simulink model "inverters_action_ETR07"  (R2017b)
settings: Solver=FixedStepAuto  StartTime=0.0  StopTime=10.0  RelTol=1e-3
libraries: simulink x8
settings Model: Creator=cspt  LastModifiedBy=cspt
settings RTWCC: SystemTargetFile=irt.tlc  TemplateMakefile=irt_default_tmf  Description=INTECRIO Real-Time Target
settings STFCustomTargetCC: TargetLangStandard=C99 (ISO)  UtilityFuncGeneration=Shared location  SystemTargetFile=irt.tlc
settings GRTTargetCC: UtilityFuncGeneration=Shared location  ParMdlRefBuildCompliant=off  CompOptLevelCompliant=off  ConcurrentExecutionCompliant=off  CombineOutputUpdateFcns=off  MatFileLogging=off  CPPClassGenCompliant=off  GRTInterface=on  UseToolchainInfoCompliant=off  GenerateASAP2=on

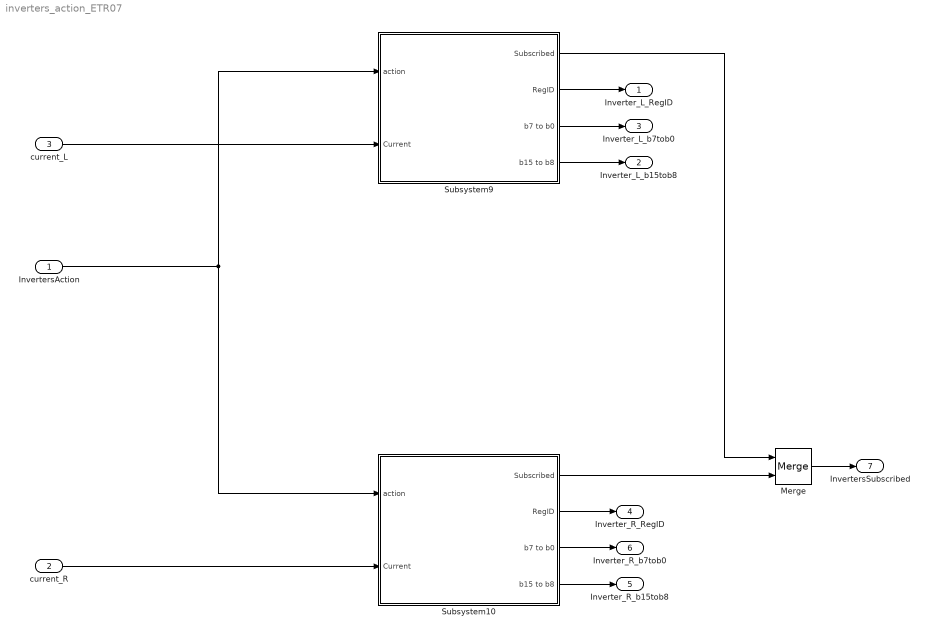
== system inverters_action_ETR07 ==
  InvertersAction : Inport
  current_R : Inport  Port=2
  current_L : Inport  Port=3
  Merge : Merge
  Subsystem10 : Subsystem
  Subsystem9 : Subsystem
  Inverter_L_RegID : Outport
  Inverter_L_b15tob8 : Outport  Port=2
  Inverter_L_b7tob0 : Outport  Port=3
  Inverter_R_RegID : Outport  Port=4
  Inverter_R_b15tob8 : Outport  Port=5
  Inverter_R_b7tob0 : Outport  Port=6
  InvertersSubscribed : Outport  Port=7
  wires:
  Subsystem9/3(b7 to b0) -> Inverter_L_b7tob0/1
  Subsystem10/1(Subscribed) -> Merge/2
  Merge/1 -> InvertersSubscribed/1
  Subsystem9/2(RegID) -> Inverter_L_RegID/1
  Subsystem9/4(b15 to b8) -> Inverter_L_b15tob8/1
  Subsystem10/3(b7 to b0) -> Inverter_R_b7tob0/1
  Subsystem10/4(b15 to b8) -> Inverter_R_b15tob8/1
  Subsystem9/1(Subscribed) -> Merge/1
  Subsystem10/2(RegID) -> Inverter_R_RegID/1
  InvertersAction/1 -> Subsystem10/1(action), Subsystem9/1(action)
  current_R/1 -> Subsystem10/2(Current)
  current_L/1 -> Subsystem9/2(Current)

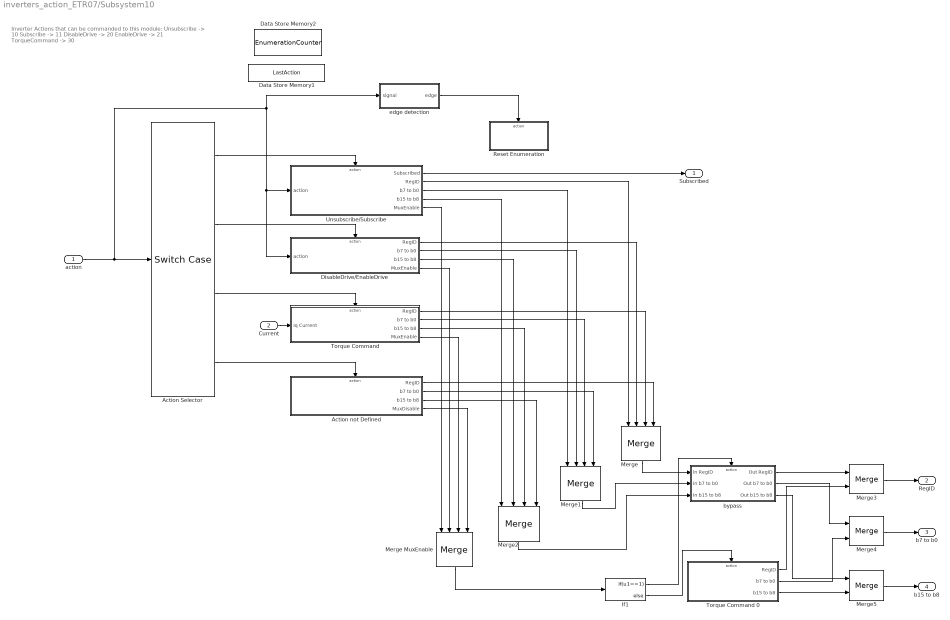
== system inverters_action_ETR07/Subsystem10 ==
  note: Inverter Actions that can be commanded to this module:
      | Unsubscribe -> 10
      | Subscribe -> 11
      |
      | DisableDrive -> 20
      | EnableDrive -> 21
      |
      | TorqueCommand -> 30
  action : Inport
  Current : Inport  Port=2
  Action Selector : SwitchCase  CaseConditions={[10,11],[20,21],30}
  Action not Defined : Subsystem
  Data Store Memory1 : DataStoreMemory  DataStoreName=LastAction  ReadBeforeWriteMsg=warning  WriteAfterWriteMsg=warning  WriteAfterReadMsg=warning  ShowAdditionalParam=off
  Data Store Memory2 : DataStoreMemory  DataStoreName=EnumerationCounter  ReadBeforeWriteMsg=warning  WriteAfterWriteMsg=warning  WriteAfterReadMsg=warning  ShowAdditionalParam=off
  DisableDrive/EnableDrive : Subsystem  TreatAsAtomicUnit=on
  If1 : If  IfExpression=u1==1
  Merge : Merge  Inputs=4
  Merge MuxEnable : Merge  Inputs=4
  Merge1 : Merge  Inputs=4
  Merge2 : Merge  Inputs=4
  Merge3 : Merge
  Merge4 : Merge
  Merge5 : Merge
  Reset Enumeration : Subsystem  TreatAsAtomicUnit=on
  Torque Command : Subsystem  TreatAsAtomicUnit=on
  Torque Command 0 : Subsystem  TreatAsAtomicUnit=on
  Unsubscribe/Subscribe : Subsystem
  bypass : Subsystem  TreatAsAtomicUnit=on
  edge detection : Subsystem
  Subscribed : Outport
  RegID : Outport  Port=2
  b7 to b0 : Outport  Port=3
  b15 to b8 : Outport  Port=4
  wires:
  Action Selector/2 -> DisableDrive/EnableDrive/Action
  Action Selector/1 -> Unsubscribe/Subscribe/Action
  Unsubscribe/Subscribe/3(b7 to b0) -> Merge1/1
  DisableDrive/EnableDrive/3(b15 to b8) -> Merge2/2
  Merge2/1 -> bypass/3(In b15 to b8)
  Unsubscribe/Subscribe/5(MuxEnable) -> Merge MuxEnable/1
  If1/2 -> Torque Command 0/Action
  DisableDrive/EnableDrive/2(b7 to b0) -> Merge1/2
  bypass/2(Out b7 to b0) -> Merge4/1
  Torque Command/3(b15 to b8) -> Merge2/3
  bypass/1(Out RegID) -> Merge3/1
  Merge1/1 -> bypass/2(In b7 to b0)
  Action not Defined/4(MuxDisable) -> Merge MuxEnable/4
  DisableDrive/EnableDrive/4(MuxEnable) -> Merge MuxEnable/2
  DisableDrive/EnableDrive/1(RegID) -> Merge/2
  Torque Command/4(MuxEnable) -> Merge MuxEnable/3
  Torque Command 0/1(RegID) -> Merge3/2
  If1/1 -> bypass/Action
  bypass/3(Out b15 to b8) -> Merge5/1
  Torque Command 0/3(b15 to b8) -> Merge5/2
  Torque Command 0/2(b7 to b0) -> Merge4/2
  Merge3/1 -> RegID/1
  Merge4/1 -> b7 to b0/1
  Torque Command/1(RegID) -> Merge/3
  Merge/1 -> bypass/1(In RegID)
  Unsubscribe/Subscribe/4(b15 to b8) -> Merge2/1
  Action Selector/3 -> Torque Command/Action
  Action Selector/4 -> Action not Defined/Action
  Merge MuxEnable/1 -> If1/1
  Torque Command/2(b7 to b0) -> Merge1/3
  Unsubscribe/Subscribe/2(RegID) -> Merge/1
  Action not Defined/2(b7 to b0) -> Merge1/4
  edge detection/1(edge) -> Reset Enumeration/Action
  action/1 -> DisableDrive/EnableDrive/1(action), Unsubscribe/Subscribe/1(action), edge detection/1(signal), Action Selector/1
  Action not Defined/1(RegID) -> Merge/4
  Unsubscribe/Subscribe/1(Subscribed) -> Subscribed/1
  Current/1 -> Torque Command/1(Iq Current)
  Action not Defined/3(b15 to b8) -> Merge2/4
  Merge5/1 -> b15 to b8/1

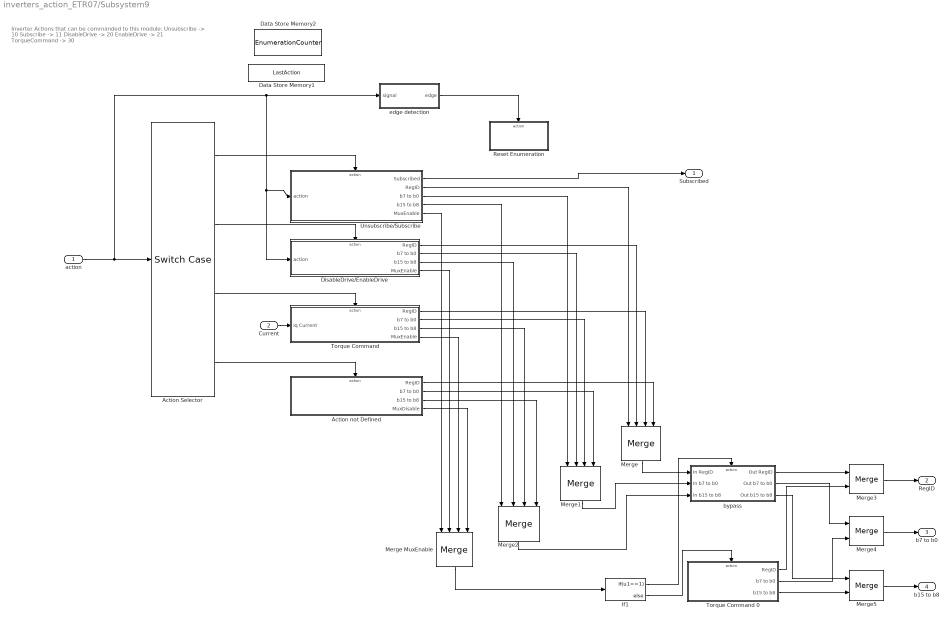
== system inverters_action_ETR07/Subsystem9 ==
  note: Inverter Actions that can be commanded to this module:
      | Unsubscribe -> 10
      | Subscribe -> 11
      |
      | DisableDrive -> 20
      | EnableDrive -> 21
      |
      | TorqueCommand -> 30
  action : Inport
  Current : Inport  Port=2
  Action Selector : SwitchCase  CaseConditions={[10,11],[20,21],30}
  Action not Defined : Subsystem
  Data Store Memory1 : DataStoreMemory  DataStoreName=LastAction  ReadBeforeWriteMsg=warning  WriteAfterWriteMsg=warning  WriteAfterReadMsg=warning  ShowAdditionalParam=off
  Data Store Memory2 : DataStoreMemory  DataStoreName=EnumerationCounter  ReadBeforeWriteMsg=warning  WriteAfterWriteMsg=warning  WriteAfterReadMsg=warning  ShowAdditionalParam=off
  DisableDrive/EnableDrive : Subsystem  TreatAsAtomicUnit=on
  If1 : If  IfExpression=u1==1
  Merge : Merge  Inputs=4
  Merge MuxEnable : Merge  Inputs=4
  Merge1 : Merge  Inputs=4
  Merge2 : Merge  Inputs=4
  Merge3 : Merge
  Merge4 : Merge
  Merge5 : Merge
  Reset Enumeration : Subsystem  TreatAsAtomicUnit=on
  Torque Command : Subsystem  TreatAsAtomicUnit=on
  Torque Command 0 : Subsystem  TreatAsAtomicUnit=on
  Unsubscribe/Subscribe : Subsystem
  bypass : Subsystem  TreatAsAtomicUnit=on
  edge detection : Subsystem
  Subscribed : Outport
  RegID : Outport  Port=2
  b7 to b0 : Outport  Port=3
  b15 to b8 : Outport  Port=4
  wires:
  Action Selector/2 -> DisableDrive/EnableDrive/Action
  Action Selector/1 -> Unsubscribe/Subscribe/Action
  Unsubscribe/Subscribe/3(b7 to b0) -> Merge1/1
  DisableDrive/EnableDrive/3(b15 to b8) -> Merge2/2
  Merge2/1 -> bypass/3(In b15 to b8)
  Unsubscribe/Subscribe/5(MuxEnable) -> Merge MuxEnable/1
  If1/2 -> Torque Command 0/Action
  DisableDrive/EnableDrive/2(b7 to b0) -> Merge1/2
  bypass/2(Out b7 to b0) -> Merge4/1
  Torque Command/3(b15 to b8) -> Merge2/3
  bypass/1(Out RegID) -> Merge3/1
  Merge1/1 -> bypass/2(In b7 to b0)
  Action not Defined/4(MuxDisable) -> Merge MuxEnable/4
  DisableDrive/EnableDrive/4(MuxEnable) -> Merge MuxEnable/2
  DisableDrive/EnableDrive/1(RegID) -> Merge/2
  Torque Command/4(MuxEnable) -> Merge MuxEnable/3
  Torque Command 0/1(RegID) -> Merge3/2
  If1/1 -> bypass/Action
  bypass/3(Out b15 to b8) -> Merge5/1
  Torque Command 0/3(b15 to b8) -> Merge5/2
  Torque Command 0/2(b7 to b0) -> Merge4/2
  Merge3/1 -> RegID/1
  Merge4/1 -> b7 to b0/1
  Torque Command/1(RegID) -> Merge/3
  Merge/1 -> bypass/1(In RegID)
  Unsubscribe/Subscribe/4(b15 to b8) -> Merge2/1
  Action Selector/3 -> Torque Command/Action
  Action Selector/4 -> Action not Defined/Action
  Merge MuxEnable/1 -> If1/1
  Torque Command/2(b7 to b0) -> Merge1/3
  Unsubscribe/Subscribe/2(RegID) -> Merge/1
  Action not Defined/2(b7 to b0) -> Merge1/4
  edge detection/1(edge) -> Reset Enumeration/Action
  action/1 -> DisableDrive/EnableDrive/1(action), Unsubscribe/Subscribe/1(action), edge detection/1(signal), Action Selector/1
  Action not Defined/1(RegID) -> Merge/4
  Unsubscribe/Subscribe/1(Subscribed) -> Subscribed/1
  Current/1 -> Torque Command/1(Iq Current)
  Action not Defined/3(b15 to b8) -> Merge2/4
  Merge5/1 -> b15 to b8/1

== system inverters_action_ETR07/Subsystem10/Action not Defined ==
  Action Port : ActionPort  ActionType=default
  "0 " : Constant  Value=0  OutDataTypeStr=boolean
  0 1 : Constant  Value=0  OutDataTypeStr=uint8
  0 2 : Constant  Value=0  OutDataTypeStr=uint8
  0 3 : Constant  Value=0  OutDataTypeStr=uint8
  RegID : Outport
  b7 to b0 : Outport  Port=2
  b15 to b8 : Outport  Port=3
  MuxDisable : Outport  Port=4
  wires:
  "0 "/1 -> MuxDisable/1
  0 1/1 -> RegID/1
  0 2/1 -> b7 to b0/1
  0 3/1 -> b15 to b8/1

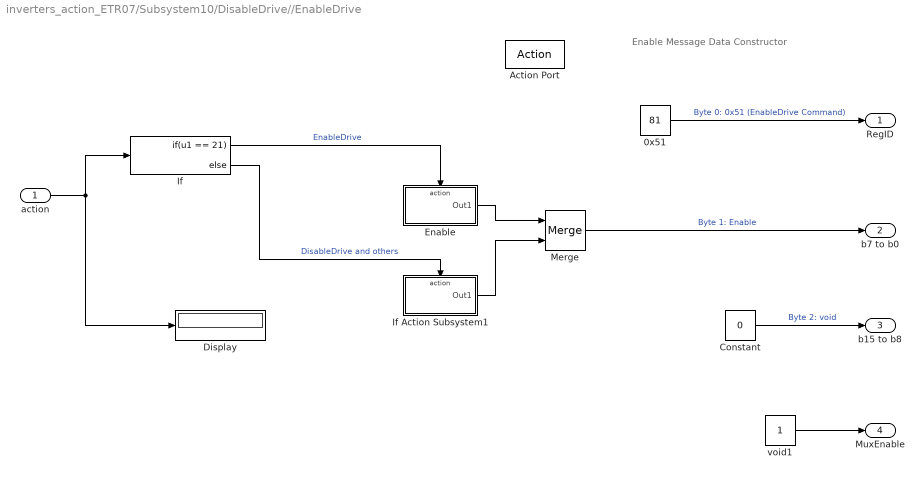
== system inverters_action_ETR07/Subsystem10/DisableDrive//EnableDrive ==
  note: Enable Message Data Constructor
  action : Inport
  Action Port : ActionPort  ActionType=case
  0x51 : Constant  Value=81  OutDataTypeStr=uint8
  Constant : Constant  Value=0  OutDataTypeStr=uint8
  Display : Display
  Enable : Subsystem  TreatAsAtomicUnit=on
  If : If  IfExpression=u1 == 21
  If Action Subsystem1 : Subsystem  TreatAsAtomicUnit=on
  Merge : Merge
  void1 : Constant  OutDataTypeStr=boolean
  RegID : Outport
  b7 to b0 : Outport  Port=2
  b15 to b8 : Outport  Port=3
  MuxEnable : Outport  Port=4
  wires:
  action/1 -> If/1, Display/1
  0x51/1 -> RegID/1  "Byte 0: 0x51 (EnableDrive Command)"
  Merge/1 -> b7 to b0/1  "Byte 1: Enable"
  void1/1 -> MuxEnable/1
  Constant/1 -> b15 to b8/1  "Byte 2: void"
  If/1 -> Enable/Action  "EnableDrive"
  If/2 -> If Action Subsystem1/Action  "DisableDrive and others"
  Enable/1(Out1) -> Merge/1
  If Action Subsystem1/1(Out1) -> Merge/2

== system inverters_action_ETR07/Subsystem10/Reset Enumeration ==
  Action Port : ActionPort  ActionType=then
  Constant1 : Constant  Value=0
  Parameter Counter Write : DataStoreWrite  DataStoreName=EnumerationCounter
  wires:
  Constant1/1 -> Parameter Counter Write/1

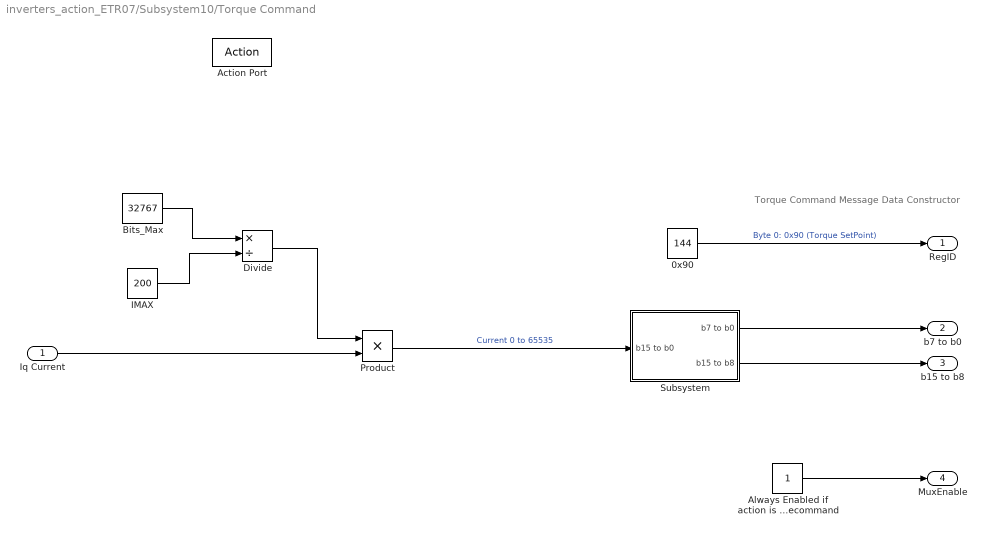
== system inverters_action_ETR07/Subsystem10/Torque Command ==
  note: Torque Command Message Data Constructor
  Iq Current : Inport
  Action Port : ActionPort  ActionType=case
  0x90 : Constant  Value=144  OutDataTypeStr=uint8
  Always Enabled if action is torquecommand : Constant  OutDataTypeStr=boolean
  Bits_Max : Constant  Value=32767
  Divide : Product  Inputs=*/
  IMAX : Constant  Value=200
  Product : Product  OutDataTypeStr=uint16
  Subsystem : Subsystem
  RegID : Outport
  b7 to b0 : Outport  Port=2
  b15 to b8 : Outport  Port=3
  MuxEnable : Outport  Port=4
  wires:
  0x90/1 -> RegID/1  "Byte 0: 0x90 (Torque SetPoint)"
  Always Enabled if action is torquecommand/1 -> MuxEnable/1
  Divide/1 -> Product/1
  Bits_Max/1 -> Divide/1
  IMAX/1 -> Divide/2
  Iq Current/1 -> Product/2
  Product/1 -> Subsystem/1(b15 to b0)  "Current 0 to 65535"
  Subsystem/1(b7 to b0) -> b7 to b0/1
  Subsystem/2(b15 to b8) -> b15 to b8/1

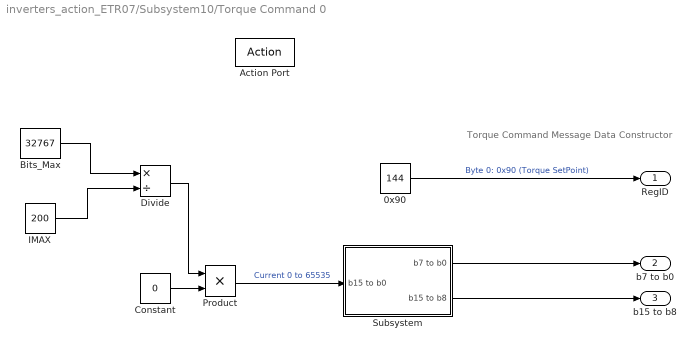
== system inverters_action_ETR07/Subsystem10/Torque Command 0 ==
  note: Torque Command Message Data Constructor
  Action Port : ActionPort  ActionType=else
  0x90 : Constant  Value=144  OutDataTypeStr=uint8
  Bits_Max : Constant  Value=32767
  Constant : Constant  Value=0
  Divide : Product  Inputs=*/
  IMAX : Constant  Value=200
  Product : Product  OutDataTypeStr=uint16
  Subsystem : Subsystem
  RegID : Outport
  b7 to b0 : Outport  Port=2
  b15 to b8 : Outport  Port=3
  wires:
  0x90/1 -> RegID/1  "Byte 0: 0x90 (Torque SetPoint)"
  Divide/1 -> Product/1
  Bits_Max/1 -> Divide/1
  IMAX/1 -> Divide/2
  Constant/1 -> Product/2
  Product/1 -> Subsystem/1(b15 to b0)  "Current 0 to 65535"
  Subsystem/1(b7 to b0) -> b7 to b0/1
  Subsystem/2(b15 to b8) -> b15 to b8/1

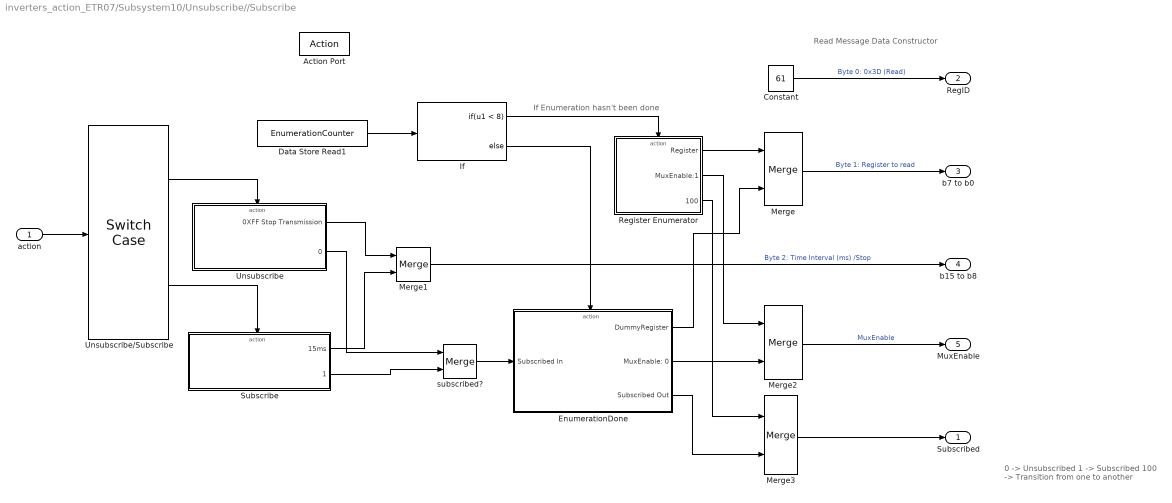
== system inverters_action_ETR07/Subsystem10/Unsubscribe//Subscribe ==
  note: 0 -> Unsubscribed
      | 1 -> Subscribed
      | 100 -> Transition from one to another
  note: Read Message Data Constructor
  note: If Enumeration hasn't been done
  action : Inport
  Action Port : ActionPort  ActionType=case
  Constant : Constant  Value=61  OutDataTypeStr=uint8
  Data Store Read1 : DataStoreRead  DataStoreName=EnumerationCounter
  EnumerationDone : Subsystem  TreatAsAtomicUnit=on
  If : If  IfExpression=u1 < 8
  Merge{,1..3} (4 alike) : Merge
  "Register Enumerator " : Subsystem  TreatAsAtomicUnit=on
  Subscribe : Subsystem  TreatAsAtomicUnit=on
  Unsubscribe : Subsystem  TreatAsAtomicUnit=on
  Unsubscribe/Subscribe : SwitchCase  CaseConditions={10,11}  ShowDefaultCase=off
  subscribed? : Merge
  Subscribed : Outport  OutDataTypeStr=boolean
  RegID : Outport  Port=2
  b7 to b0 : Outport  Port=3  OutDataTypeStr=uint8
  b15 to b8 : Outport  Port=4  OutDataTypeStr=uint8
  MuxEnable : Outport  Port=5  OutDataTypeStr=boolean
  wires:
  If/1 -> "Register Enumerator "/Action
  "Register Enumerator "/1(Register) -> Merge/1
  Constant/1 -> RegID/1  "Byte 0: 0x3D (Read)"
  Merge1/1 -> b15 to b8/1  "Byte 2: Time Interval (ms) /Stop"
  Unsubscribe/Subscribe/1 -> Unsubscribe/Action
  Unsubscribe/Subscribe/2 -> Subscribe/Action
  EnumerationDone/1(DummyRegister) -> Merge/2
  If/2 -> EnumerationDone/Action
  Merge/1 -> b7 to b0/1  "Byte 1: Register to read"
  action/1 -> Unsubscribe/Subscribe/1
  Unsubscribe/1(0XFF Stop Transmission) -> Merge1/1
  Subscribe/1(15ms) -> Merge1/2
  EnumerationDone/2(MuxEnable: 0) -> Merge2/2
  "Register Enumerator "/2(MuxEnable:1) -> Merge2/1
  Merge2/1 -> MuxEnable/1  "MuxEnable"
  Data Store Read1/1 -> If/1
  Unsubscribe/2(0) -> subscribed?/1
  Subscribe/2(1) -> subscribed?/2
  subscribed?/1 -> EnumerationDone/1(Subscribed In)
  "Register Enumerator "/3(100) -> Merge3/1
  EnumerationDone/3(Subscribed Out) -> Merge3/2
  Merge3/1 -> Subscribed/1

== system inverters_action_ETR07/Subsystem10/bypass ==
  In RegID : Inport
  In b7 to b0 : Inport  Port=2
  In b15 to b8 : Inport  Port=3
  Action Port : ActionPort  ActionType=then
  Out RegID : Outport
  Out b7 to b0 : Outport  Port=2  OutDataTypeStr=uint8
  Out b15 to b8 : Outport  Port=3  OutDataTypeStr=uint8
  wires:
  In RegID/1 -> Out RegID/1
  In b7 to b0/1 -> Out b7 to b0/1
  In b15 to b8/1 -> Out b15 to b8/1

== system inverters_action_ETR07/Subsystem10/edge detection ==
  signal : Inport
  Delay : Delay  DelayLength=1
  If2 : If  NumInputs=2  IfExpression=u1 ~= u2  ShowElse=off
  edge : Outport
  wires:
  signal/1 -> Delay/1, If2/1
  If2/1 -> edge/1  "if action this is a new action"
  Delay/1 -> If2/2

== system inverters_action_ETR07/Subsystem9/Action not Defined ==
  Action Port : ActionPort  ActionType=default
  "0 " : Constant  Value=0  OutDataTypeStr=boolean
  0 1 : Constant  Value=0  OutDataTypeStr=uint8
  0 2 : Constant  Value=0  OutDataTypeStr=uint8
  0 3 : Constant  Value=0  OutDataTypeStr=uint8
  RegID : Outport
  b7 to b0 : Outport  Port=2
  b15 to b8 : Outport  Port=3
  MuxDisable : Outport  Port=4
  wires:
  "0 "/1 -> MuxDisable/1
  0 1/1 -> RegID/1
  0 2/1 -> b7 to b0/1
  0 3/1 -> b15 to b8/1

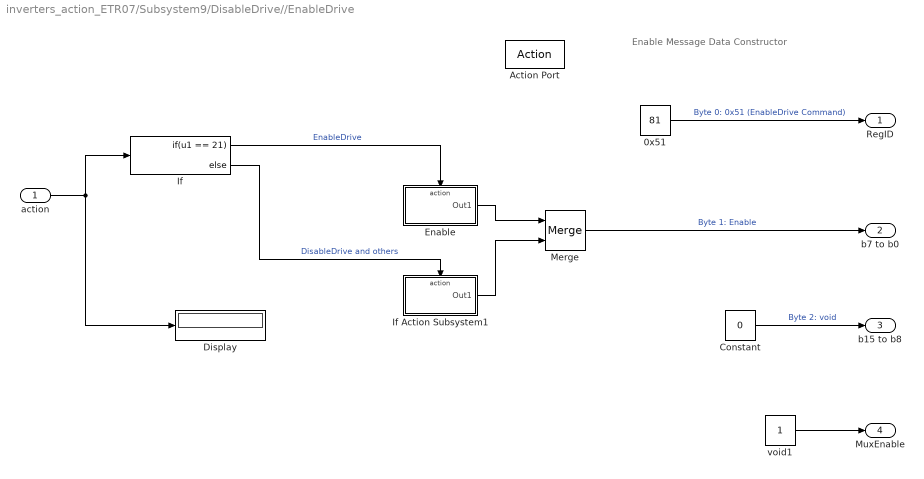
== system inverters_action_ETR07/Subsystem9/DisableDrive//EnableDrive ==
  note: Enable Message Data Constructor
  action : Inport
  Action Port : ActionPort  ActionType=case
  0x51 : Constant  Value=81  OutDataTypeStr=uint8
  Constant : Constant  Value=0  OutDataTypeStr=uint8
  Display : Display
  Enable : Subsystem  TreatAsAtomicUnit=on
  If : If  IfExpression=u1 == 21
  If Action Subsystem1 : Subsystem  TreatAsAtomicUnit=on
  Merge : Merge
  void1 : Constant  OutDataTypeStr=boolean
  RegID : Outport
  b7 to b0 : Outport  Port=2
  b15 to b8 : Outport  Port=3
  MuxEnable : Outport  Port=4
  wires:
  action/1 -> If/1, Display/1
  0x51/1 -> RegID/1  "Byte 0: 0x51 (EnableDrive Command)"
  Merge/1 -> b7 to b0/1  "Byte 1: Enable"
  void1/1 -> MuxEnable/1
  Constant/1 -> b15 to b8/1  "Byte 2: void"
  If/1 -> Enable/Action  "EnableDrive"
  If/2 -> If Action Subsystem1/Action  "DisableDrive and others"
  Enable/1(Out1) -> Merge/1
  If Action Subsystem1/1(Out1) -> Merge/2

== system inverters_action_ETR07/Subsystem9/Reset Enumeration ==
  Action Port : ActionPort  ActionType=then
  Constant1 : Constant  Value=0
  Parameter Counter Write : DataStoreWrite  DataStoreName=EnumerationCounter
  wires:
  Constant1/1 -> Parameter Counter Write/1

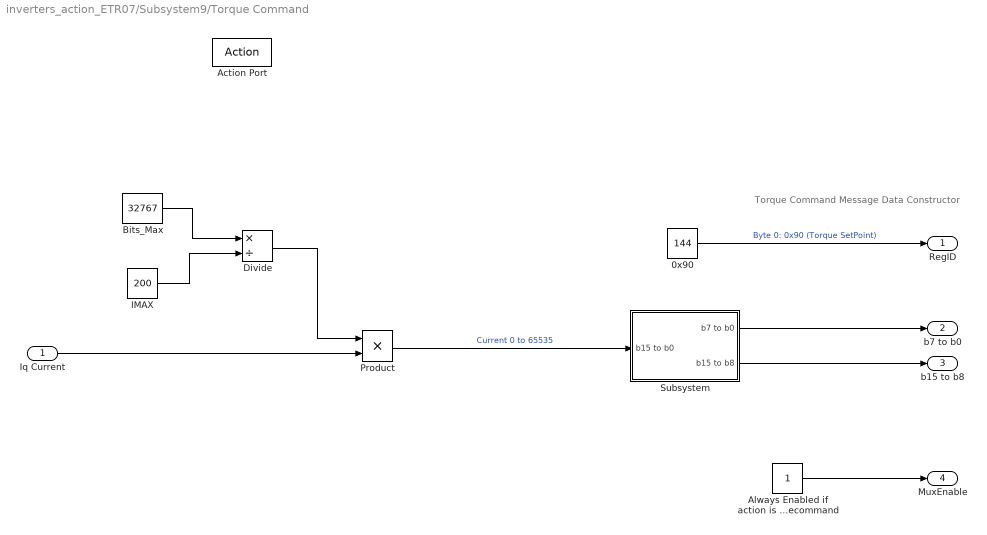
== system inverters_action_ETR07/Subsystem9/Torque Command ==
  note: Torque Command Message Data Constructor
  Iq Current : Inport
  Action Port : ActionPort  ActionType=case
  0x90 : Constant  Value=144  OutDataTypeStr=uint8
  Always Enabled if action is torquecommand : Constant  OutDataTypeStr=boolean
  Bits_Max : Constant  Value=32767
  Divide : Product  Inputs=*/
  IMAX : Constant  Value=200
  Product : Product  OutDataTypeStr=uint16
  Subsystem : Subsystem
  RegID : Outport
  b7 to b0 : Outport  Port=2
  b15 to b8 : Outport  Port=3
  MuxEnable : Outport  Port=4
  wires:
  0x90/1 -> RegID/1  "Byte 0: 0x90 (Torque SetPoint)"
  Always Enabled if action is torquecommand/1 -> MuxEnable/1
  Divide/1 -> Product/1
  Bits_Max/1 -> Divide/1
  IMAX/1 -> Divide/2
  Iq Current/1 -> Product/2
  Product/1 -> Subsystem/1(b15 to b0)  "Current 0 to 65535"
  Subsystem/1(b7 to b0) -> b7 to b0/1
  Subsystem/2(b15 to b8) -> b15 to b8/1

== system inverters_action_ETR07/Subsystem9/Torque Command 0 ==
  note: Torque Command Message Data Constructor
  Action Port : ActionPort  ActionType=else
  0x90 : Constant  Value=144  OutDataTypeStr=uint8
  Bits_Max : Constant  Value=32767
  Constant : Constant  Value=0
  Divide : Product  Inputs=*/
  IMAX : Constant  Value=200
  Product : Product  OutDataTypeStr=uint16
  Subsystem : Subsystem
  RegID : Outport
  b7 to b0 : Outport  Port=2
  b15 to b8 : Outport  Port=3
  wires:
  0x90/1 -> RegID/1  "Byte 0: 0x90 (Torque SetPoint)"
  Divide/1 -> Product/1
  Bits_Max/1 -> Divide/1
  IMAX/1 -> Divide/2
  Constant/1 -> Product/2
  Product/1 -> Subsystem/1(b15 to b0)  "Current 0 to 65535"
  Subsystem/1(b7 to b0) -> b7 to b0/1
  Subsystem/2(b15 to b8) -> b15 to b8/1

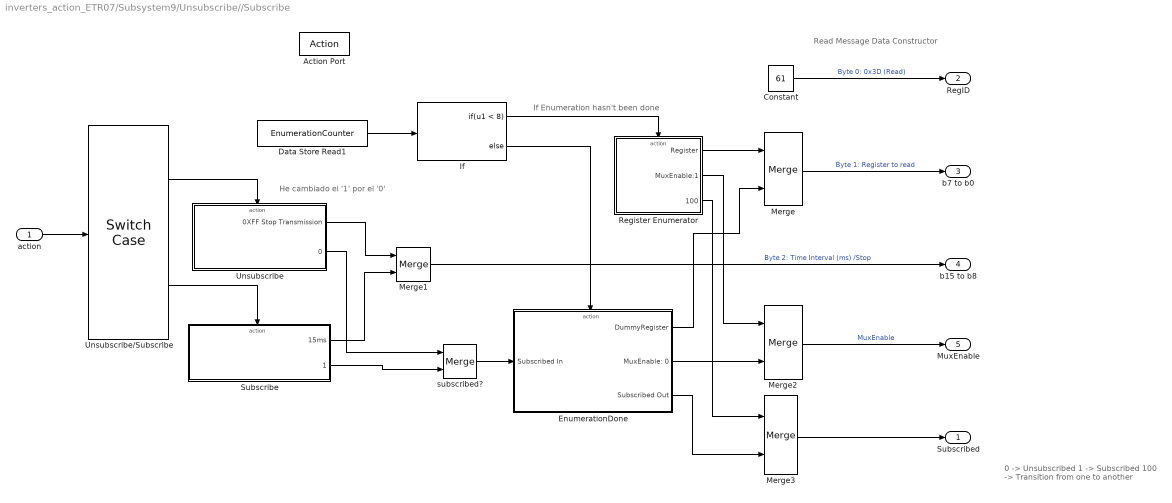
== system inverters_action_ETR07/Subsystem9/Unsubscribe//Subscribe ==
  note: He cambiado el '1' por el '0'
  note: 0 -> Unsubscribed
      | 1 -> Subscribed
      | 100 -> Transition from one to another
  note: Read Message Data Constructor
  note: If Enumeration hasn't been done
  action : Inport
  Action Port : ActionPort  ActionType=case
  Constant : Constant  Value=61  OutDataTypeStr=uint8
  Data Store Read1 : DataStoreRead  DataStoreName=EnumerationCounter
  EnumerationDone : Subsystem  TreatAsAtomicUnit=on
  If : If  IfExpression=u1 < 8
  Merge{,1..3} (4 alike) : Merge
  "Register Enumerator " : Subsystem  TreatAsAtomicUnit=on
  Subscribe : Subsystem  TreatAsAtomicUnit=on
  Unsubscribe : Subsystem  TreatAsAtomicUnit=on
  Unsubscribe/Subscribe : SwitchCase  CaseConditions={10,11}  ShowDefaultCase=off
  subscribed? : Merge
  Subscribed : Outport  OutDataTypeStr=boolean
  RegID : Outport  Port=2
  b7 to b0 : Outport  Port=3  OutDataTypeStr=uint8
  b15 to b8 : Outport  Port=4  OutDataTypeStr=uint8
  MuxEnable : Outport  Port=5  OutDataTypeStr=boolean
  wires:
  If/1 -> "Register Enumerator "/Action
  "Register Enumerator "/1(Register) -> Merge/1
  Constant/1 -> RegID/1  "Byte 0: 0x3D (Read)"
  Merge1/1 -> b15 to b8/1  "Byte 2: Time Interval (ms) /Stop"
  Unsubscribe/Subscribe/1 -> Unsubscribe/Action
  Unsubscribe/Subscribe/2 -> Subscribe/Action
  EnumerationDone/1(DummyRegister) -> Merge/2
  If/2 -> EnumerationDone/Action
  Merge/1 -> b7 to b0/1  "Byte 1: Register to read"
  action/1 -> Unsubscribe/Subscribe/1
  Unsubscribe/1(0XFF Stop Transmission) -> Merge1/1
  Subscribe/1(15ms) -> Merge1/2
  EnumerationDone/2(MuxEnable: 0) -> Merge2/2
  "Register Enumerator "/2(MuxEnable:1) -> Merge2/1
  Merge2/1 -> MuxEnable/1  "MuxEnable"
  Data Store Read1/1 -> If/1
  Unsubscribe/2(0) -> subscribed?/1
  subscribed?/1 -> EnumerationDone/1(Subscribed In)
  "Register Enumerator "/3(100) -> Merge3/1
  EnumerationDone/3(Subscribed Out) -> Merge3/2
  Merge3/1 -> Subscribed/1
  Subscribe/2(1) -> subscribed?/2

== system inverters_action_ETR07/Subsystem9/bypass ==
  In RegID : Inport
  In b7 to b0 : Inport  Port=2
  In b15 to b8 : Inport  Port=3
  Action Port : ActionPort  ActionType=then
  Out RegID : Outport
  Out b7 to b0 : Outport  Port=2  OutDataTypeStr=uint8
  Out b15 to b8 : Outport  Port=3  OutDataTypeStr=uint8
  wires:
  In RegID/1 -> Out RegID/1
  In b7 to b0/1 -> Out b7 to b0/1
  In b15 to b8/1 -> Out b15 to b8/1

== system inverters_action_ETR07/Subsystem9/edge detection ==
  signal : Inport
  Delay : Delay  DelayLength=1
  If2 : If  NumInputs=2  IfExpression=u1 ~= u2  ShowElse=off
  edge : Outport
  wires:
  signal/1 -> Delay/1, If2/1
  If2/1 -> edge/1  "if action this is a new action"
  Delay/1 -> If2/2

== system inverters_action_ETR07/Subsystem10/DisableDrive//EnableDrive/Enable ==
  Action Port : ActionPort  ActionType=then
  Constant : Constant  Value=0  OutDataTypeStr=uint8  SampleTime=-1
  Out1 : Outport
  wires:
  Constant/1 -> Out1/1

== system inverters_action_ETR07/Subsystem10/DisableDrive//EnableDrive/If Action Subsystem1 ==
  Action Port : ActionPort  ActionType=else
  Constant : Constant  Value=4  OutDataTypeStr=uint8
  Out1 : Outport
  wires:
  Constant/1 -> Out1/1

== system inverters_action_ETR07/Subsystem10/Torque Command/Subsystem ==
  b15 to b0 : Inport
  Bitwise Operator : simulink/Logic and Bit Operations/Bitwise Operator  logicop=AND  UseBitMask=on  BitMask='00FF'  BitMaskRealWorld=Stored Integer
  Bitwise Operator1 : simulink/Logic and Bit Operations/Bitwise Operator  logicop=AND  UseBitMask=on  BitMask='00FF'  BitMaskRealWorld=Stored Integer
  Data Type Conversion : DataTypeConversion  OutDataTypeStr=uint8
  Data Type Conversion1 : DataTypeConversion  OutDataTypeStr=uint8
  Shift Arithmetic : ArithShift  BitShiftNumber=8
  b7 to b0 : Outport  OutDataTypeStr=uint8
  b15 to b8 : Outport  Port=2  OutDataTypeStr=uint8
  wires:
  Data Type Conversion1/1 -> b15 to b8/1
  Data Type Conversion/1 -> b7 to b0/1
  Bitwise Operator/1 -> Data Type Conversion/1  "b7 to b0"
  Shift Arithmetic/1 -> Bitwise Operator1/1
  Bitwise Operator1/1 -> Data Type Conversion1/1
  b15 to b0/1 -> Shift Arithmetic/1, Bitwise Operator/1

== system inverters_action_ETR07/Subsystem10/Torque Command 0/Subsystem ==
  b15 to b0 : Inport
  Bitwise Operator : simulink/Logic and Bit Operations/Bitwise Operator  logicop=AND  UseBitMask=on  BitMask='00FF'  BitMaskRealWorld=Stored Integer
  Bitwise Operator1 : simulink/Logic and Bit Operations/Bitwise Operator  logicop=AND  UseBitMask=on  BitMask='00FF'  BitMaskRealWorld=Stored Integer
  Data Type Conversion : DataTypeConversion  OutDataTypeStr=uint8
  Data Type Conversion1 : DataTypeConversion  OutDataTypeStr=uint8
  Shift Arithmetic : ArithShift  BitShiftNumber=8
  b7 to b0 : Outport  OutDataTypeStr=uint8
  b15 to b8 : Outport  Port=2  OutDataTypeStr=uint8
  wires:
  Data Type Conversion1/1 -> b15 to b8/1
  Data Type Conversion/1 -> b7 to b0/1
  Bitwise Operator/1 -> Data Type Conversion/1  "b7 to b0"
  Shift Arithmetic/1 -> Bitwise Operator1/1
  Bitwise Operator1/1 -> Data Type Conversion1/1
  b15 to b0/1 -> Shift Arithmetic/1, Bitwise Operator/1

== system inverters_action_ETR07/Subsystem10/Unsubscribe//Subscribe/EnumerationDone ==
  Subscribed In : Inport
  Action Port : ActionPort  ActionType=else
  Constant : Constant  Value=0  OutDataTypeStr=uint8
  Constant1 : Constant  Value=0  OutDataTypeStr=boolean
  DummyRegister : Outport
  MuxEnable: 0 : Outport  Port=2
  Subscribed Out : Outport  Port=3  OutDataTypeStr=boolean
  wires:
  Constant/1 -> DummyRegister/1
  Constant1/1 -> MuxEnable: 0/1
  Subscribed In/1 -> Subscribed Out/1

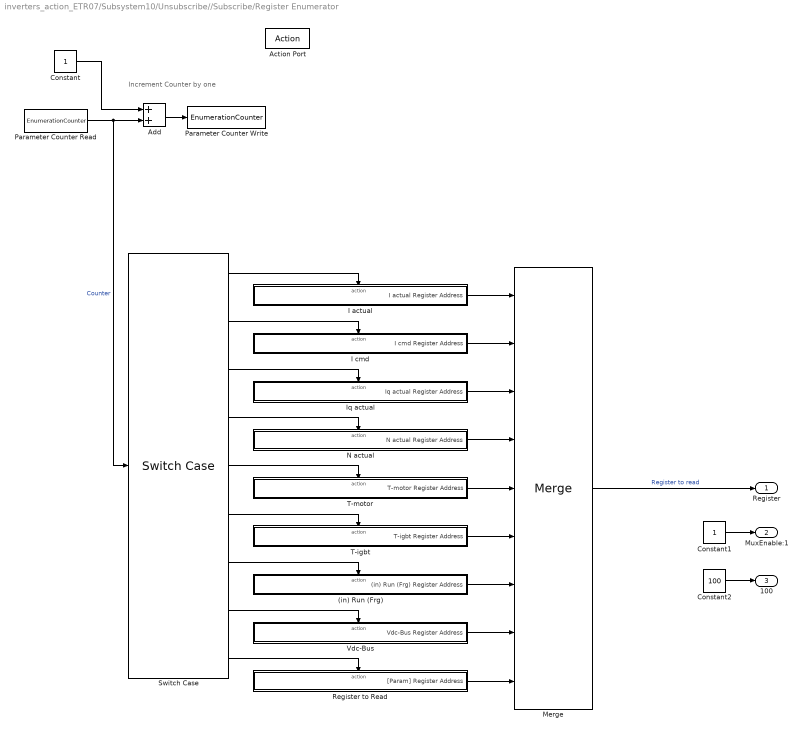
== system inverters_action_ETR07/Subsystem10/Unsubscribe//Subscribe/Register Enumerator  ==
  note: Increment Counter by one
  Action Port : ActionPort  ActionType=then
  (in) Run (Frg) : Subsystem  TreatAsAtomicUnit=on
  Add : Sum
  Constant : Constant
  Constant1 : Constant  OutDataTypeStr=boolean
  Constant2 : Constant  Value=100  OutDataTypeStr=boolean
  I actual : Subsystem  TreatAsAtomicUnit=on
  I cmd : Subsystem  TreatAsAtomicUnit=on
  Iq actual : Subsystem  TreatAsAtomicUnit=on
  Merge : Merge  Inputs=9
  N actual : Subsystem  TreatAsAtomicUnit=on
  Parameter Counter Read : DataStoreRead  DataStoreName=EnumerationCounter
  Parameter Counter Write : DataStoreWrite  DataStoreName=EnumerationCounter
  Register to Read : Subsystem  TreatAsAtomicUnit=on
  Switch Case : SwitchCase  CaseConditions={0,1,2,3,4,5,6,7}
  T-igbt : Subsystem  TreatAsAtomicUnit=on
  T-motor : Subsystem  TreatAsAtomicUnit=on
  Vdc-Bus : Subsystem  TreatAsAtomicUnit=on
  Register : Outport
  MuxEnable:1 : Outport  Port=2
  100 : Outport  Port=3  OutDataTypeStr=boolean
  wires:
  Parameter Counter Read/1 -> Add/2, Switch Case/1  "Counter"
  Add/1 -> Parameter Counter Write/1
  Constant/1 -> Add/1
  Switch Case/1 -> I actual/Action
  Switch Case/9 -> Register to Read/Action
  Switch Case/2 -> I cmd/Action
  Switch Case/3 -> Iq actual/Action
  Switch Case/4 -> N actual/Action
  Switch Case/6 -> T-igbt/Action
  Switch Case/7 -> (in) Run (Frg)/Action
  I actual/1(I actual Register Address) -> Merge/1
  I cmd/1(I cmd Register Address) -> Merge/2
  Iq actual/1(Iq actual Register Address) -> Merge/3
  N actual/1(N actual Register Address) -> Merge/4
  T-motor/1(T-motor Register Address) -> Merge/5
  T-igbt/1(T-igbt Register Address) -> Merge/6
  (in) Run (Frg)/1((in) Run (Frg) Register Address) -> Merge/7
  Vdc-Bus/1(Vdc-Bus Register Address) -> Merge/8
  Register to Read/1("[Param] Register Address") -> Merge/9
  Merge/1 -> Register/1  "Register to read"
  Constant1/1 -> MuxEnable:1/1
  Constant2/1 -> 100/1
  Switch Case/8 -> Vdc-Bus/Action
  Switch Case/5 -> T-motor/Action

== system inverters_action_ETR07/Subsystem10/Unsubscribe//Subscribe/Subscribe ==
  Action Port : ActionPort  ActionType=case
  " " : Constant  OutDataTypeStr=boolean
  Time Interval : Constant  Value=25  OutDataTypeStr=uint8
  15ms : Outport
  1 : Outport  Port=2
  wires:
  Time Interval/1 -> 15ms/1
  " "/1 -> 1/1

== system inverters_action_ETR07/Subsystem10/Unsubscribe//Subscribe/Unsubscribe ==
  Action Port : ActionPort  ActionType=case
  " " : Constant  Value=0  OutDataTypeStr=boolean
  0XFF : Constant  Value=255  OutDataTypeStr=uint8
  0XFF Stop Transmission : Outport
  0 : Outport  Port=2
  wires:
  0XFF/1 -> 0XFF Stop Transmission/1
  " "/1 -> 0/1

== system inverters_action_ETR07/Subsystem9/DisableDrive//EnableDrive/Enable ==
  Action Port : ActionPort  ActionType=then
  Constant : Constant  Value=0  OutDataTypeStr=uint8  SampleTime=-1
  Out1 : Outport
  wires:
  Constant/1 -> Out1/1

== system inverters_action_ETR07/Subsystem9/DisableDrive//EnableDrive/If Action Subsystem1 ==
  Action Port : ActionPort  ActionType=else
  Constant : Constant  Value=4  OutDataTypeStr=uint8
  Out1 : Outport
  wires:
  Constant/1 -> Out1/1

== system inverters_action_ETR07/Subsystem9/Torque Command/Subsystem ==
  b15 to b0 : Inport
  Bitwise Operator : simulink/Logic and Bit Operations/Bitwise Operator  logicop=AND  UseBitMask=on  BitMask='00FF'  BitMaskRealWorld=Stored Integer
  Bitwise Operator1 : simulink/Logic and Bit Operations/Bitwise Operator  logicop=AND  UseBitMask=on  BitMask='00FF'  BitMaskRealWorld=Stored Integer
  Data Type Conversion : DataTypeConversion  OutDataTypeStr=uint8
  Data Type Conversion1 : DataTypeConversion  OutDataTypeStr=uint8
  Shift Arithmetic : ArithShift  BitShiftNumber=8
  b7 to b0 : Outport  OutDataTypeStr=uint8
  b15 to b8 : Outport  Port=2  OutDataTypeStr=uint8
  wires:
  Data Type Conversion1/1 -> b15 to b8/1
  Data Type Conversion/1 -> b7 to b0/1
  Bitwise Operator/1 -> Data Type Conversion/1  "b7 to b0"
  Shift Arithmetic/1 -> Bitwise Operator1/1
  Bitwise Operator1/1 -> Data Type Conversion1/1
  b15 to b0/1 -> Shift Arithmetic/1, Bitwise Operator/1

== system inverters_action_ETR07/Subsystem9/Torque Command 0/Subsystem ==
  b15 to b0 : Inport
  Bitwise Operator : simulink/Logic and Bit Operations/Bitwise Operator  logicop=AND  UseBitMask=on  BitMask='00FF'  BitMaskRealWorld=Stored Integer
  Bitwise Operator1 : simulink/Logic and Bit Operations/Bitwise Operator  logicop=AND  UseBitMask=on  BitMask='00FF'  BitMaskRealWorld=Stored Integer
  Data Type Conversion : DataTypeConversion  OutDataTypeStr=uint8
  Data Type Conversion1 : DataTypeConversion  OutDataTypeStr=uint8
  Shift Arithmetic : ArithShift  BitShiftNumber=8
  b7 to b0 : Outport  OutDataTypeStr=uint8
  b15 to b8 : Outport  Port=2  OutDataTypeStr=uint8
  wires:
  Data Type Conversion1/1 -> b15 to b8/1
  Data Type Conversion/1 -> b7 to b0/1
  Bitwise Operator/1 -> Data Type Conversion/1  "b7 to b0"
  Shift Arithmetic/1 -> Bitwise Operator1/1
  Bitwise Operator1/1 -> Data Type Conversion1/1
  b15 to b0/1 -> Shift Arithmetic/1, Bitwise Operator/1

== system inverters_action_ETR07/Subsystem9/Unsubscribe//Subscribe/EnumerationDone ==
  Subscribed In : Inport
  Action Port : ActionPort  ActionType=else
  Constant : Constant  Value=0  OutDataTypeStr=uint8
  Constant1 : Constant  Value=0  OutDataTypeStr=boolean
  DummyRegister : Outport
  MuxEnable: 0 : Outport  Port=2
  Subscribed Out : Outport  Port=3  OutDataTypeStr=boolean
  wires:
  Constant/1 -> DummyRegister/1
  Constant1/1 -> MuxEnable: 0/1
  Subscribed In/1 -> Subscribed Out/1

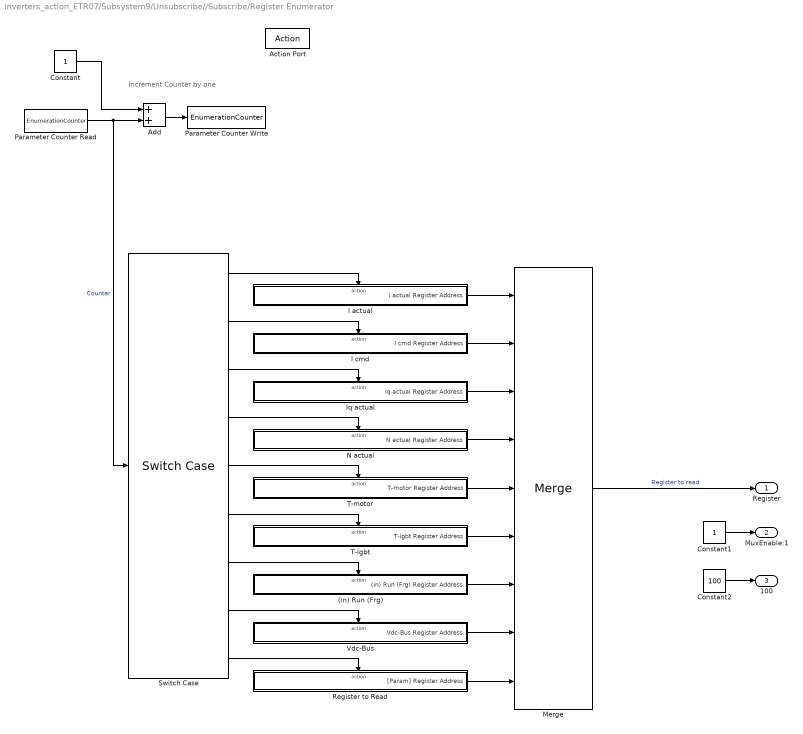
== system inverters_action_ETR07/Subsystem9/Unsubscribe//Subscribe/Register Enumerator  ==
  note: Increment Counter by one
  Action Port : ActionPort  ActionType=then
  (in) Run (Frg) : Subsystem  TreatAsAtomicUnit=on
  Add : Sum
  Constant : Constant
  Constant1 : Constant  OutDataTypeStr=boolean
  Constant2 : Constant  Value=100  OutDataTypeStr=boolean
  I actual : Subsystem  TreatAsAtomicUnit=on
  I cmd : Subsystem  TreatAsAtomicUnit=on
  Iq actual : Subsystem  TreatAsAtomicUnit=on
  Merge : Merge  Inputs=9
  N actual : Subsystem  TreatAsAtomicUnit=on
  Parameter Counter Read : DataStoreRead  DataStoreName=EnumerationCounter
  Parameter Counter Write : DataStoreWrite  DataStoreName=EnumerationCounter
  Register to Read : Subsystem  TreatAsAtomicUnit=on
  Switch Case : SwitchCase  CaseConditions={0,1,2,3,4,5,6,7}
  T-igbt : Subsystem  TreatAsAtomicUnit=on
  T-motor : Subsystem  TreatAsAtomicUnit=on
  Vdc-Bus : Subsystem  TreatAsAtomicUnit=on
  Register : Outport
  MuxEnable:1 : Outport  Port=2
  100 : Outport  Port=3  OutDataTypeStr=boolean
  wires:
  Parameter Counter Read/1 -> Add/2, Switch Case/1  "Counter"
  Add/1 -> Parameter Counter Write/1
  Constant/1 -> Add/1
  Switch Case/1 -> I actual/Action
  Switch Case/9 -> Register to Read/Action
  Switch Case/2 -> I cmd/Action
  Switch Case/3 -> Iq actual/Action
  Switch Case/4 -> N actual/Action
  Switch Case/6 -> T-igbt/Action
  Switch Case/7 -> (in) Run (Frg)/Action
  I actual/1(I actual Register Address) -> Merge/1
  I cmd/1(I cmd Register Address) -> Merge/2
  Iq actual/1(Iq actual Register Address) -> Merge/3
  N actual/1(N actual Register Address) -> Merge/4
  T-motor/1(T-motor Register Address) -> Merge/5
  T-igbt/1(T-igbt Register Address) -> Merge/6
  (in) Run (Frg)/1((in) Run (Frg) Register Address) -> Merge/7
  Vdc-Bus/1(Vdc-Bus Register Address) -> Merge/8
  Register to Read/1("[Param] Register Address") -> Merge/9
  Merge/1 -> Register/1  "Register to read"
  Constant1/1 -> MuxEnable:1/1
  Constant2/1 -> 100/1
  Switch Case/8 -> Vdc-Bus/Action
  Switch Case/5 -> T-motor/Action

== system inverters_action_ETR07/Subsystem9/Unsubscribe//Subscribe/Subscribe ==
  Action Port : ActionPort  ActionType=case
  " 1" : Constant  OutDataTypeStr=boolean
  Time Interval : Constant  Value=25  OutDataTypeStr=uint8
  15ms : Outport
  1 : Outport  Port=2
  wires:
  Time Interval/1 -> 15ms/1
  " 1"/1 -> 1/1

== system inverters_action_ETR07/Subsystem9/Unsubscribe//Subscribe/Unsubscribe ==
  Action Port : ActionPort  ActionType=case
  " " : Constant  OutDataTypeStr=boolean
  0XFF : Constant  Value=255  OutDataTypeStr=uint8
  0XFF Stop Transmission : Outport
  0 : Outport  Port=2
  wires:
  0XFF/1 -> 0XFF Stop Transmission/1
  " "/1 -> 0/1

== system inverters_action_ETR07/Subsystem10/Unsubscribe//Subscribe/Register Enumerator /(in) Run (Frg) ==
  note: this constant is the register adress converted into decimal value
  Action Port : ActionPort  ActionType=case
  0xE8 : Constant  Value=232  OutDataTypeStr=uint8
  (in) Run (Frg) Register Address : Outport
  wires:
  0xE8/1 -> (in) Run (Frg) Register Address/1

== system inverters_action_ETR07/Subsystem10/Unsubscribe//Subscribe/Register Enumerator /I actual ==
  note: this constant is the register address converted into decimal value
  Action Port : ActionPort  ActionType=case
  0x20 : Constant  Value=32  OutDataTypeStr=uint8
  I actual Register Address : Outport
  wires:
  0x20/1 -> I actual Register Address/1

== system inverters_action_ETR07/Subsystem10/Unsubscribe//Subscribe/Register Enumerator /I cmd ==
  note: this constant is the register adress converted into decimal value
  Action Port : ActionPort  ActionType=case
  0x26 : Constant  Value=38  OutDataTypeStr=uint8
  I cmd Register Address : Outport
  wires:
  0x26/1 -> I cmd Register Address/1

== system inverters_action_ETR07/Subsystem10/Unsubscribe//Subscribe/Register Enumerator /Iq actual ==
  note: this constant is the register adress converted into decimal value
  Action Port : ActionPort  ActionType=case
  0x27 : Constant  Value=39  OutDataTypeStr=uint8
  Iq actual Register Address : Outport
  wires:
  0x27/1 -> Iq actual Register Address/1

== system inverters_action_ETR07/Subsystem10/Unsubscribe//Subscribe/Register Enumerator /N actual ==
  note: this constant is the register adress converted into decimal value
  Action Port : ActionPort  ActionType=case
  0x30 : Constant  Value=48  OutDataTypeStr=uint8
  N actual Register Address : Outport
  wires:
  0x30/1 -> N actual Register Address/1

== system inverters_action_ETR07/Subsystem10/Unsubscribe//Subscribe/Register Enumerator /Register to Read ==
  note: this constant is the register adress converted into decimal value
  Action Port : ActionPort  ActionType=default
  " Register adress" : Constant  Value=0  OutDataTypeStr=uint8
  "[Param] Register Address" : Outport
  wires:
  " Register adress"/1 -> "[Param] Register Address"/1

== system inverters_action_ETR07/Subsystem10/Unsubscribe//Subscribe/Register Enumerator /T-igbt ==
  note: this constant is the register adress converted into decimal value
  Action Port : ActionPort  ActionType=case
  0x4A : Constant  Value=74  OutDataTypeStr=uint8
  T-igbt Register Address : Outport
  wires:
  0x4A/1 -> T-igbt Register Address/1

== system inverters_action_ETR07/Subsystem10/Unsubscribe//Subscribe/Register Enumerator /T-motor ==
  note: this constant is the register adress converted into decimal value
  Action Port : ActionPort  ActionType=case
  0x49 : Constant  Value=73  OutDataTypeStr=uint8
  T-motor Register Address : Outport
  wires:
  0x49/1 -> T-motor Register Address/1

== system inverters_action_ETR07/Subsystem10/Unsubscribe//Subscribe/Register Enumerator /Vdc-Bus ==
  note: this constant is the register adress converted into decimal value
  Action Port : ActionPort  ActionType=case
  0xEB : Constant  Value=235  OutDataTypeStr=uint8
  Vdc-Bus Register Address : Outport
  wires:
  0xEB/1 -> Vdc-Bus Register Address/1

== system inverters_action_ETR07/Subsystem9/Unsubscribe//Subscribe/Register Enumerator /(in) Run (Frg) ==
  note: this constant is the register adress converted into decimal value
  Action Port : ActionPort
  0xE8 : Constant  Value=232  OutDataTypeStr=uint8
  (in) Run (Frg) Register Address : Outport
  wires:
  0xE8/1 -> (in) Run (Frg) Register Address/1

== system inverters_action_ETR07/Subsystem9/Unsubscribe//Subscribe/Register Enumerator /I actual ==
  note: this constant is the register address converted into decimal value
  Action Port : ActionPort
  0x20 : Constant  Value=32  OutDataTypeStr=uint8
  I actual Register Address : Outport
  wires:
  0x20/1 -> I actual Register Address/1

== system inverters_action_ETR07/Subsystem9/Unsubscribe//Subscribe/Register Enumerator /I cmd ==
  note: this constant is the register adress converted into decimal value
  Action Port : ActionPort
  0x26 : Constant  Value=38  OutDataTypeStr=uint8
  I cmd Register Address : Outport
  wires:
  0x26/1 -> I cmd Register Address/1

== system inverters_action_ETR07/Subsystem9/Unsubscribe//Subscribe/Register Enumerator /Iq actual ==
  note: this constant is the register adress converted into decimal value
  Action Port : ActionPort
  0x27 : Constant  Value=39  OutDataTypeStr=uint8
  Iq actual Register Address : Outport
  wires:
  0x27/1 -> Iq actual Register Address/1

== system inverters_action_ETR07/Subsystem9/Unsubscribe//Subscribe/Register Enumerator /N actual ==
  note: this constant is the register adress converted into decimal value
  Action Port : ActionPort
  0x30 : Constant  Value=48  OutDataTypeStr=uint8
  N actual Register Address : Outport
  wires:
  0x30/1 -> N actual Register Address/1

== system inverters_action_ETR07/Subsystem9/Unsubscribe//Subscribe/Register Enumerator /Register to Read ==
  note: this constant is the register adress converted into decimal value
  Action Port : ActionPort
  " Register adress" : Constant  Value=0  OutDataTypeStr=uint8
  "[Param] Register Address" : Outport
  wires:
  " Register adress"/1 -> "[Param] Register Address"/1

== system inverters_action_ETR07/Subsystem9/Unsubscribe//Subscribe/Register Enumerator /T-igbt ==
  note: this constant is the register adress converted into decimal value
  Action Port : ActionPort
  0x4A : Constant  Value=74  OutDataTypeStr=uint8
  T-igbt Register Address : Outport
  wires:
  0x4A/1 -> T-igbt Register Address/1

== system inverters_action_ETR07/Subsystem9/Unsubscribe//Subscribe/Register Enumerator /T-motor ==
  note: this constant is the register adress converted into decimal value
  Action Port : ActionPort
  0x49 : Constant  Value=73  OutDataTypeStr=uint8
  T-motor Register Address : Outport
  wires:
  0x49/1 -> T-motor Register Address/1

== system inverters_action_ETR07/Subsystem9/Unsubscribe//Subscribe/Register Enumerator /Vdc-Bus ==
  note: this constant is the register adress converted into decimal value
  Action Port : ActionPort
  0xEB : Constant  Value=235  OutDataTypeStr=uint8
  Vdc-Bus Register Address : Outport
  wires:
  0xEB/1 -> Vdc-Bus Register Address/1
